simulink model "prob_7"  (R2020b)
settings: Solver=VariableStepAuto  StartTime=0.0  StopTime=10.0  RelTol=1e-3
values from neighbouring files (symbols this model uses):
  a0 = 1    [Initializing_prob7.m]
  a1 = 1    [Initializing_prob7.m]
  a2 = -1    [Initializing_prob7.m]
  b0 = 1    [Initializing_prob7.m]
  b1 = 2    [Initializing_prob7.m]
  b2 = -1    [Initializing_prob7.m]
settings Model: Creator=Lakshmi  LastModifiedBy=Lakshmi

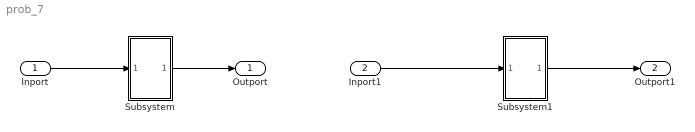
== system prob_7 ==
  Inport : Inport
  Inport1 : Inport  Port=2
  Subsystem : Subsystem
  Subsystem1 : Subsystem
  Outport : Outport
  Outport1 : Outport  Port=2
  wires:
  Inport/1 -> Subsystem/1(In1)
  Subsystem/1(Out1) -> Outport/1
  Inport1/1 -> Subsystem1/1(In1)
  Subsystem1/1(Out1) -> Outport1/1

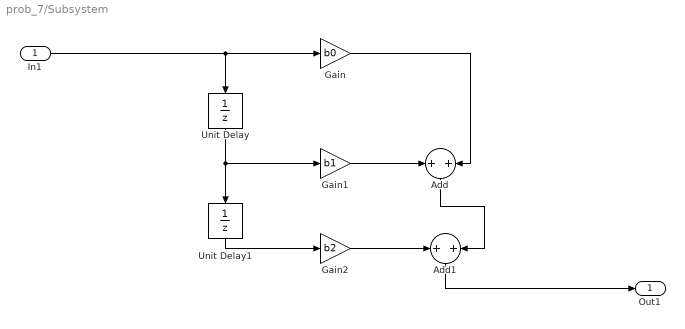
== system prob_7/Subsystem ==
  In1 : Inport
  Add : Sum
  Add1 : Sum
  Gain : Gain  Gain=b0
  Gain1 : Gain  Gain=b1
  Gain2 : Gain  Gain=b2
  Unit Delay : UnitDelay  SampleTime=-1  HasFrameUpgradeWarning=on
  Unit Delay1 : UnitDelay  SampleTime=-1  HasFrameUpgradeWarning=on
  Out1 : Outport
  wires:
  Unit Delay1/1 -> Gain2/1
  Unit Delay/1 -> Unit Delay1/1, Gain1/1
  Add/1 -> Add1/2
  Gain1/1 -> Add/1
  Gain2/1 -> Add1/1
  In1/1 -> Unit Delay/1, Gain/1
  Gain/1 -> Add/2
  Add1/1 -> Out1/1

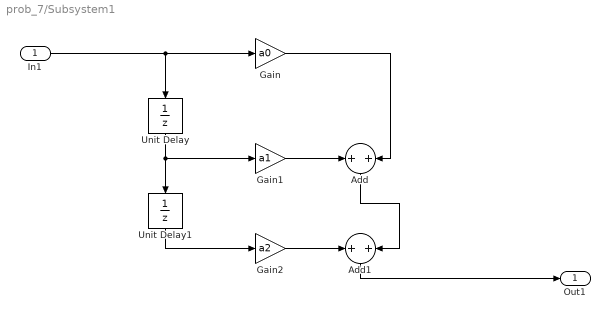
== system prob_7/Subsystem1 ==
  In1 : Inport
  Add : Sum
  Add1 : Sum
  Gain : Gain  Gain=a0
  Gain1 : Gain  Gain=a1
  Gain2 : Gain  Gain=a2
  Unit Delay : UnitDelay  SampleTime=-1  HasFrameUpgradeWarning=on
  Unit Delay1 : UnitDelay  SampleTime=-1  HasFrameUpgradeWarning=on
  Out1 : Outport
  wires:
  Unit Delay1/1 -> Gain2/1
  Gain1/1 -> Add/1
  Add/1 -> Add1/2
  Gain/1 -> Add/2
  Gain2/1 -> Add1/1
  Unit Delay/1 -> Gain1/1, Unit Delay1/1
  Add1/1 -> Out1/1
  In1/1 -> Unit Delay/1, Gain/1
